simulink model "VertauschungssatzIntegratorTransferfunction"  (R2021b)
settings: Solver=VariableStepAuto  StartTime=0.0  StopTime=10.0  RelTol=1e-3
settings Model: Creator=PM  LastModifiedBy=PM

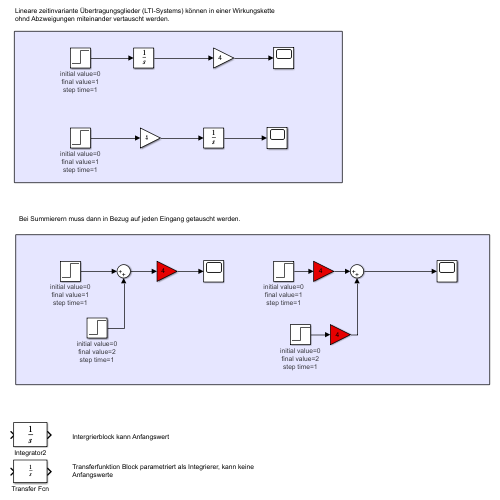
[thumbnail: Simulink's stored preview of the top-level diagram]
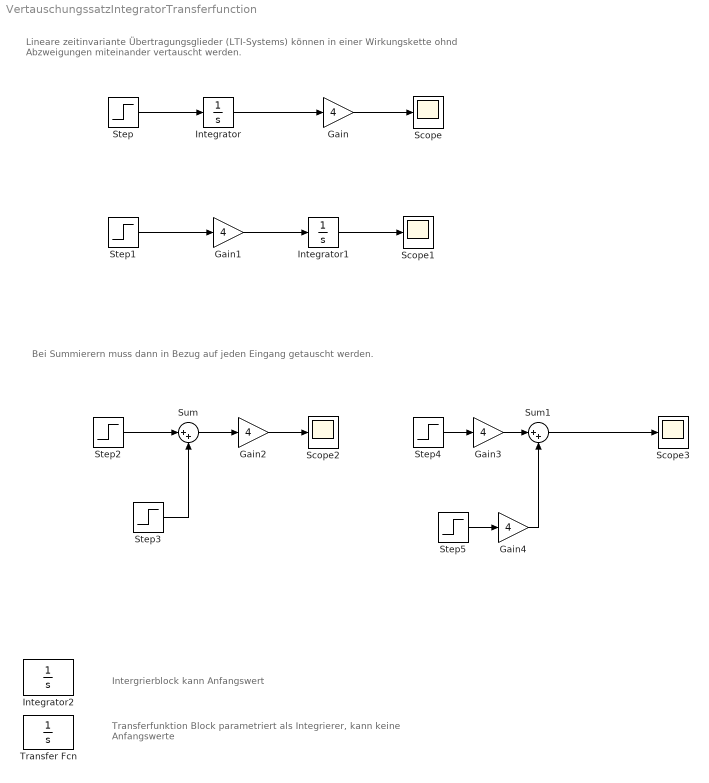
== system VertauschungssatzIntegratorTransferfunction ==
  note: Transferfunktion Block parametriert als Integrierer, kann keine
      | Anfangswerte
  note: Intergrierblock kann Anfangswert
  note: Bei Summierern muss dann in Bezug auf jeden Eingang getauscht werden.
  note: Lineare zeitinvariante Übertragungsglieder (LTI-Systems) können in einer Wirkungskette ohnd Abzweigungen miteinander vertauscht werden.
  Gain{,1..4} (5 alike) : Gain  Gain=4
  Integrator : Integrator
  Integrator1 : Integrator
  Integrator2 : Integrator
  Scope{,1..3} (4 alike) : Scope
  Step{,1..2,4} (4 alike) : Step  SampleTime=0
      settings: AttributesFormatString=initial value=%<Before>\nfinal value=%<After>\nstep time=%<Time>
  Step3 : Step  After=2  SampleTime=0
      settings: AttributesFormatString=initial value=%<Before>\nfinal value=%<After>\nstep time=%<Time>
  Step5 : Step  After=2  SampleTime=0
      settings: AttributesFormatString=initial value=%<Before>\nfinal value=%<After>\nstep time=%<Time>
  Sum : Sum  Inputs=|++
  Sum1 : Sum  Inputs=|++
  Transfer Fcn : TransferFcn  Numerator=[1 ]  Denominator=[1 0]
  wires:
  Step/1 -> Integrator/1
  Integrator/1 -> Gain/1
  Gain/1 -> Scope/1
  Step1/1 -> Gain1/1
  Gain1/1 -> Integrator1/1
  Integrator1/1 -> Scope1/1
  Step2/1 -> Sum/1
  Step3/1 -> Sum/2
  Sum/1 -> Gain2/1
  Gain2/1 -> Scope2/1
  Gain3/1 -> Sum1/1
  Step4/1 -> Gain3/1
  Step5/1 -> Gain4/1
  Gain4/1 -> Sum1/2
  Sum1/1 -> Scope3/1
